simulink model "Control_Simulink"  (R2013a)
settings: Solver=ode45  StartTime=0.0  StopTime=10.0  RelTol=1e-3
undefined symbols (not defined in the file): b, k, m
settings Model: Creator=B407  LastModifiedBy=B407

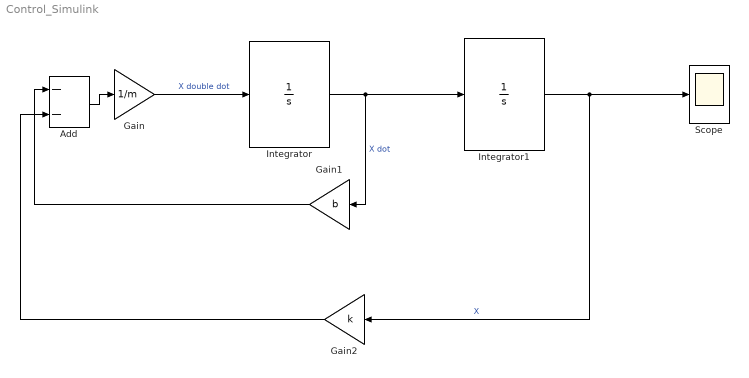
== system Control_Simulink ==
  Add : Sum  Inputs=--
  Gain : Gain  Gain=1/m
  Gain1 : Gain  Gain=b
  Gain2 : Gain  Gain=k
  Integrator : Integrator  InitialCondition=10
  Integrator1 : Integrator  InitialCondition=10
  Scope : Scope
  wires:
  Integrator/1 -> Gain1/1, Integrator1/1  "X dot"
  Gain/1 -> Integrator/1  "X double dot"
  Integrator1/1 -> Scope/1, Gain2/1  "X"
  Add/1 -> Gain/1
  Gain1/1 -> Add/1
  Gain2/1 -> Add/2
